simulink model "radarSim4"  (R2023b)
settings: Solver=FixedStepAuto  StartTime=0.0  StopTime=simTime  RelTol=1e-3
values from neighbouring files (symbols this model uses):
  c = get(groot,'defaultAxesColorOrder')    [compareData.m]
undefined symbols (not defined in the file or in its folder): fs, txDf_Dt, windowLen
libraries: dspsrcs4 x3, dspstat3 x2, paullib x2, hdlsllib x1
settings Model: Creator=pbroo  LastModifiedBy=pbroo
settings SolverCC: AutoInsertRateTranBlk=on
settings OptimizationCC: BlockReduction=off  ConditionallyExecuteInputs=off  DefaultParameterBehavior=Inlined
settings DebuggingCC: AlgebraicLoopMsg=error  SingleTaskRateTransMsg=error
settings HardwareCC: ProdBitPerPointer=32  ProdBitPerSizeT=32  ProdBitPerPtrDiffT=32  ProdLargestAtomicFloat=None  ProdIntDivRoundTo=Undefined  ProdEndianess=Unspecified  ProdWordSize=32  ProdHWDeviceType=ASIC/FPGA->ASIC/FPGA  TargetBitPerPointer=64  TargetBitPerSizeT=64  TargetBitPerPtrDiffT=64  TargetLongLongMode=on  TargetIntDivRoundTo=Zero  TargetEndianess=LittleEndian  TargetWordSize=64  TargetHWDeviceType=Custom Processor->MATLAB Host Computer  ProdEqTarget=off

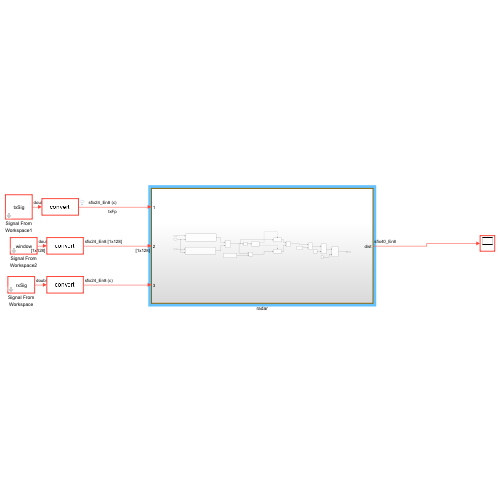
[thumbnail: Simulink's stored preview of the top-level diagram]
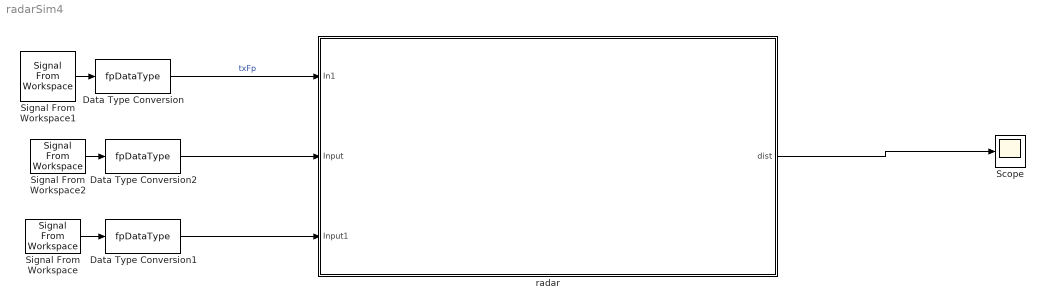
== system radarSim4 ==
  Data Type Conversion : DataTypeConversion  OutDataTypeStr=fpDataType  SaturateOnIntegerOverflow=off  RndMeth=Floor
  Data Type Conversion1 : DataTypeConversion  OutDataTypeStr=fpDataType  SaturateOnIntegerOverflow=off  RndMeth=Floor
  Data Type Conversion2 : DataTypeConversion  OutDataTypeStr=fpDataType  SaturateOnIntegerOverflow=off  RndMeth=Floor
  Scope : Scope
  Signal From Workspace : dspsrcs4/Signal From Workspace  X=rxSig  Ts=1  nsamps=1  OutputAfterFinalValue=Setting to zero  ignoreOrWarnInputAndFrameLengths=off  OutputFrames=off
  Signal From Workspace1 : dspsrcs4/Signal From Workspace  X=txSig  Ts=1  nsamps=1  OutputAfterFinalValue=Setting to zero  ignoreOrWarnInputAndFrameLengths=off  OutputFrames=off
  Signal From Workspace2 : dspsrcs4/Signal From Workspace  X=window  Ts=1  nsamps=1  OutputAfterFinalValue=Setting to zero  ignoreOrWarnInputAndFrameLengths=off  OutputFrames=off
  radar : Subsystem
  wires:
  Signal From Workspace1/1 -> Data Type Conversion/1
  Signal From Workspace/1 -> Data Type Conversion1/1
  radar/1(dist) -> Scope/1
  Data Type Conversion/1 -> radar/1(In1)  "txFp"
  Data Type Conversion1/1 -> radar/3(Input1)
  Signal From Workspace2/1 -> Data Type Conversion2/1
  Data Type Conversion2/1 -> radar/2(Input)

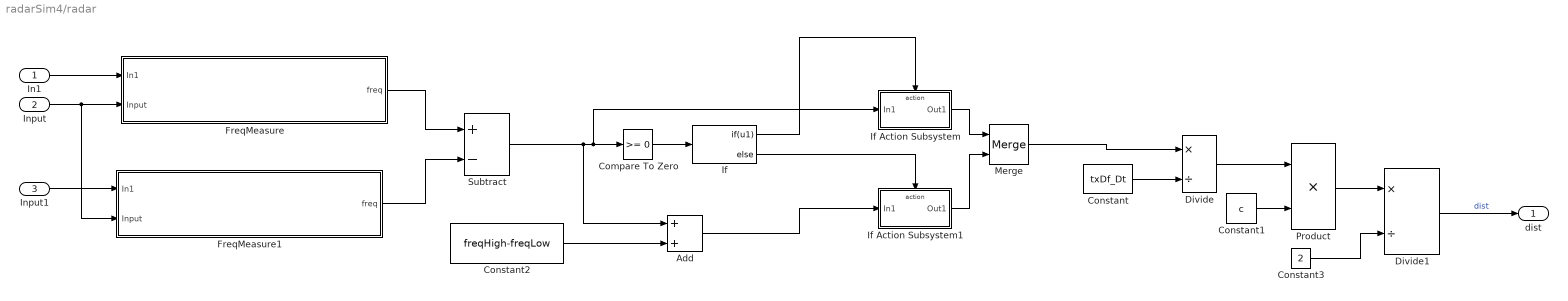
== system radarSim4/radar ==
  In1 : Inport
  Input : Inport  Port=2
  Input1 : Inport  Port=3
  Add : Sum  OutDataTypeStr=Inherit: Same as first input
  Compare To Zero : hdlsllib/Logic and Bit Operations/Compare To Zero  relop=>=  OutDataTypeStr=boolean
  Constant : Constant  Value=txDf_Dt  OutDataTypeStr=int16  SampleTime=-1
  Constant1 : Constant  Value=c  OutDataTypeStr=int16  SampleTime=-1
  Constant2 : Constant  Value=freqHigh-freqLow  OutDataTypeStr=fpDataType  SampleTime=-1
  Constant3 : Constant  Value=2  VectorParams1D=off  OutDataTypeStr=int16  SampleTime=-1
  Divide : Product  Inputs=*/  RndMeth=Simplest  SaturateOnIntegerOverflow=on
  Divide1 : Product  Inputs=*/  RndMeth=Simplest  SaturateOnIntegerOverflow=on  LockScale=on
  FreqMeasure : Subsystem
  FreqMeasure1 : Subsystem
  If : If  IfExpression=u1
  If Action Subsystem : Subsystem  TreatAsAtomicUnit=on
  If Action Subsystem1 : Subsystem  TreatAsAtomicUnit=on
  Merge : Merge
  Product : Product
  Subtract : Sum  Inputs=+-  OutDataTypeStr=fpDataType
  dist : Outport
  wires:
  FreqMeasure1/1(freq) -> Subtract/2
  Constant/1 -> Divide/2
  Divide/1 -> Product/1
  Constant1/1 -> Product/2
  FreqMeasure/1(freq) -> Subtract/1
  In1/1 -> FreqMeasure/1(In1)
  Product/1 -> Divide1/1
  Divide1/1 -> dist/1  "dist"
  Constant3/1 -> Divide1/2
  Constant2/1 -> Add/2
  Subtract/1 -> Compare To Zero/1, If Action Subsystem/1(In1), Add/1
  If/1 -> If Action Subsystem/Action
  If/2 -> If Action Subsystem1/Action
  Merge/1 -> Divide/1
  Add/1 -> If Action Subsystem1/1(In1)
  If Action Subsystem1/1(Out1) -> Merge/2
  If Action Subsystem/1(Out1) -> Merge/1
  Compare To Zero/1 -> If/1
  Input/1 -> FreqMeasure1/2(Input), FreqMeasure/2(Input)
  Input1/1 -> FreqMeasure1/1(In1)

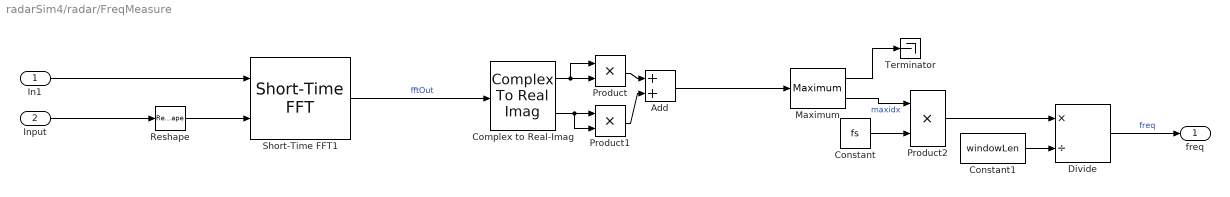
== system radarSim4/radar/FreqMeasure ==
  In1 : Inport
  Input : Inport  Port=2
  Add : Sum
  Complex to Real-Imag : ComplexToRealImag
  Constant : Constant  Value=fs  OutDataTypeStr=fpDataType  SampleTime=-1
  Constant1 : Constant  Value=windowLen  OutDataTypeStr=fpDataType  SampleTime=-1
  Divide : Product  Inputs=*/  RndMeth=Simplest  SaturateOnIntegerOverflow=on  LockScale=on
  Maximum : dspstat3/Maximum  operation=maximum  fcn=Value and Index  indexBase=One  operateOver=Each column  Dimension=1  InputProcessing=Columns as channels (frame based)  reset=None  roiEnable=off  roiType=Rectangles  roiPortion=Entire ROI  roiOutput=Individual statistics for each ROI  roiFlag=off  roundingMode=Floor  overflowMode=off  accumDataTypeStr=Inherit: Same as product output  accumLastDataTypeStr=Inherit: Same as product output
  Product : Product
  Product1 : Product
  Product2 : Product
  Reshape : Reshape  OutputDimensionality=Column vector (2-D)
  Short-Time FFT1 : paullib/Short-Time FFT  W=windowLen  OvLap=nOverlap  M=windowLen
  Terminator : Terminator
  freq : Outport
  wires:
  Maximum/2 -> Product2/1  "maxidx"
  Add/1 -> Maximum/1
  Constant1/1 -> Divide/2
  Constant/1 -> Product2/2
  Product2/1 -> Divide/1
  Divide/1 -> freq/1  "freq"
  Maximum/1 -> Terminator/1
  Short-Time FFT1/1 -> Complex to Real-Imag/1  "fftOut"
  In1/1 -> Short-Time FFT1/1
  Complex to Real-Imag/1 -> Product/1, Product/2
  Complex to Real-Imag/2 -> Product1/2, Product1/1
  Product/1 -> Add/1
  Product1/1 -> Add/2
  Reshape/1 -> Short-Time FFT1/2
  Input/1 -> Reshape/1

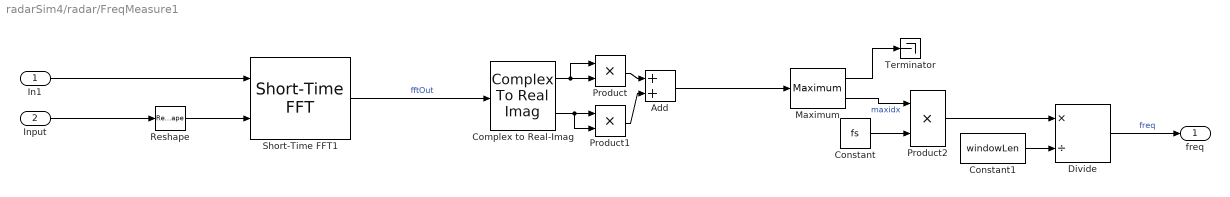
== system radarSim4/radar/FreqMeasure1 ==
  In1 : Inport
  Input : Inport  Port=2
  Add : Sum
  Complex to Real-Imag : ComplexToRealImag
  Constant : Constant  Value=fs  OutDataTypeStr=fpDataType  SampleTime=-1
  Constant1 : Constant  Value=windowLen  OutDataTypeStr=fpDataType  SampleTime=-1
  Divide : Product  Inputs=*/  RndMeth=Simplest  SaturateOnIntegerOverflow=on  LockScale=on
  Maximum : dspstat3/Maximum  operation=maximum  fcn=Value and Index  indexBase=One  operateOver=Each column  Dimension=1  InputProcessing=Columns as channels (frame based)  reset=None  roiEnable=off  roiType=Rectangles  roiPortion=Entire ROI  roiOutput=Individual statistics for each ROI  roiFlag=off  roundingMode=Floor  overflowMode=off  accumDataTypeStr=Inherit: Same as product output  accumLastDataTypeStr=Inherit: Same as product output
  Product : Product
  Product1 : Product
  Product2 : Product
  Reshape : Reshape  OutputDimensionality=Column vector (2-D)
  Short-Time FFT1 : paullib/Short-Time FFT  W=windowLen  OvLap=nOverlap  M=windowLen
  Terminator : Terminator
  freq : Outport
  wires:
  Maximum/2 -> Product2/1  "maxidx"
  Add/1 -> Maximum/1
  Constant1/1 -> Divide/2
  Constant/1 -> Product2/2
  Product2/1 -> Divide/1
  Divide/1 -> freq/1  "freq"
  Maximum/1 -> Terminator/1
  Short-Time FFT1/1 -> Complex to Real-Imag/1  "fftOut"
  In1/1 -> Short-Time FFT1/1
  Complex to Real-Imag/1 -> Product/1, Product/2
  Complex to Real-Imag/2 -> Product1/2, Product1/1
  Product/1 -> Add/1
  Product1/1 -> Add/2
  Reshape/1 -> Short-Time FFT1/2
  Input/1 -> Reshape/1

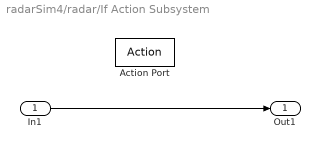
== system radarSim4/radar/If Action Subsystem ==
  In1 : Inport
  Action Port : ActionPort  ActionPortLabel=if(u1)
  Out1 : Outport  InitialOutput=0
  wires:
  In1/1 -> Out1/1

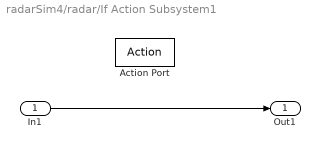
== system radarSim4/radar/If Action Subsystem1 ==
  In1 : Inport
  Action Port : ActionPort  ActionPortLabel=else
  Out1 : Outport
  wires:
  In1/1 -> Out1/1
